simulink model "DBX_model_all"  (R2015a)
settings: Solver=ode2  SolverMode=SingleTasking  StartTime=0.0  StopTime=10.0  FixedStep=T_sim  RelTol=1e-3
values from neighbouring files (symbols this model uses):
  A_M = 2/sqrt(3)*L_M    [SetupComplete.m]    (also in simple_all.m = single(A_M))
  Alpha_unique_rad = deg2rad(Alpha_unique)    [DBX_aero_V1.m]    (also in simple_all.m = single(Alpha_unique_rad))
  as = aerosonde_data_mod    [SetupComplete.m]
  B_span = 3    [SetupComplete.m]    (also in simple_all.m = single(B_span))
  Beta_unique_rad = deg2rad(Beta_unique)    [DBX_aero_V1.m]    (also in simple_all.m = single(Beta_unique_rad))
  C_D_q = 0.0336    [DBX_aero_V1.m]    (also in simple_all.m = single(C_D_q))
  C_l = NaN*ones(size(Alpha_unique,1),size(Beta_unique,1) )    [DBX_aero_V1.m]    (also in simple_all.m = single(C_l))
  C_l_delta_a_Asim = C_l_raw(idx)/deg2rad(delta_ale(idx))    [DBX_aero_V1.m]    (also in simple_all.m = single(C_l_delta_a_Asim))
  C_l_delta_rv_Asim = C_l_raw(idx)/deg2rad(delta_rud(idx))    [DBX_aero_V1.m]    (also in simple_all.m = single(C_l_delta_rv_Asim))
  C_l_p = -0.8333    [DBX_aero_V1.m]    (also in simple_all.m = single(C_l_p))
  C_l_r = 0.0347    [DBX_aero_V1.m]    (also in simple_all.m = single(C_l_r))
  C_Lift_q = 10.9    [DBX_aero_V1.m]    (also in simple_all.m = single(C_Lift_q))
  C_m = NaN*ones(size(Alpha_unique,1),size(Beta_unique,1),size(delta_elev_unique,1) )    [DBX_aero_V1.m]    (also in simple_all.m = single(C_m))
  C_m_q = -45.7828    [DBX_aero_V1.m]    (also in simple_all.m = single(C_m_q))
  C_n = NaN*ones(size(Alpha_unique,1),size(Beta_unique,1) )    [DBX_aero_V1.m]    (also in simple_all.m = single(C_n))
  C_n_delta_a_Asim = C_n_raw(idx)/deg2rad(delta_ale(idx))    [DBX_aero_V1.m]    (also in simple_all.m = single(C_n_delta_a_Asim))
  C_n_delta_rv_Asim = C_n_raw(idx)/deg2rad(delta_rud(idx))    [DBX_aero_V1.m]    (also in simple_all.m = single(C_n_delta_rv_Asim))
  C_n_p = -0.0066    [DBX_aero_V1.m]    (also in simple_all.m = single(C_n_p))
  C_n_r = -0.1827    [DBX_aero_V1.m]    (also in simple_all.m = single(C_n_r))
  C_X = NaN*ones(size(Alpha_unique,1),size(Beta_unique,1),size(delta_elev_unique,1) )    [DBX_aero_V1.m]    (also in simple_all.m = single(C_X))
  C_Y = NaN*ones(size(Alpha_unique,1),size(Beta_unique,1) )    [DBX_aero_V1.m]    (also in simple_all.m = single(C_Y))
  C_Y_delta_rv_Asim = C_y(idx)/deg2rad(delta_rud(idx))    [DBX_aero_V1.m]    (also in simple_all.m = single(C_Y_delta_rv_Asim))
  C_Y_p = -0.0991    [DBX_aero_V1.m]    (also in simple_all.m = single(C_Y_p))
  C_Y_r = 0.5219    [DBX_aero_V1.m]    (also in simple_all.m = single(C_Y_r))
  C_Z = NaN*ones(size(Alpha_unique,1),size(Beta_unique,1),size(delta_elev_unique,1) )    [DBX_aero_V1.m]    (also in simple_all.m = single(C_Z))
  CG = (m_OE*CG_OE + m_PL*CG_PL)/m    [SetupComplete.m]    (also in simple_all.m = single(CG))
  CMA = 0.25    [SetupComplete.m]    (also in simple_all.m = single(CMA))
  delta_elev_unique_rad = deg2rad(delta_elev_unique)    [DBX_aero_V1.m]    (also in simple_all.m = single(delta_elev_unique_rad))
  g = 9.81    [SetupComplete.m]    (also in simple_all.m = single(g))
  h_1 = -0.0666    [SetupComplete.m]    (also in simple_all.m = single(h_1))
  h_2 = -0.0666    [SetupComplete.m]    (also in simple_all.m = single(h_2))
  h_3 = -0.04824    [SetupComplete.m]    (also in simple_all.m = single(h_3))
  I_BAC = I_CG + m*[CG(3)^2,0,CG(1)*CG(3);0,CG(1)^2+CG(3)^2,0;CG(1)*CG(3),0,CG(1)^2]    [SetupComplete.m]    (also in simple_all.m = single(I_BAC))
  Initial_Omegas = max(0,Omega_0)    [Run_DBX.m]    (also in simple_all.m = single(Initial_Omegas))
  Initial_Torques = Torque_0    [Run_DBX.m]    (also in simple_all.m = single(Initial_Torques))
  L_M = 1.20    (= 1.2)    [SetupComplete.m]    (also in simple_all.m = single(L_M))
  m = m_OE + m_PL    (= 14.5)    [SetupComplete.m]    (also in simple_all.m = single(m))
  Rotation_sign = [-1,-1,-1]    [SetupComplete.m]    (also in simple_all.m = single(Rotation_sign))
undefined symbols (not defined in the file or in its folder): DOWN_0, EAST_0, F, MIL, NORTH_0, P_0, Q_0, R_0, Servo_calib, U_0, V_0, W_0
libraries: DBX_model x14, aerolibwind2 x6, aerolibasang x5, aerolibadyn x2, aerolibtransform2 x1
(part 1 of 2)
settings Model: ExtModeTrigDuration=5000  Creator=DavidTorres  LastModifiedBy=David
settings DataIOCC: LimitDataPoints=off  SaveOutput=off  SignalLogging=off  DSMLogging=off  VisualizeSimOutput=off  SaveTime=off
settings OptimizationCC: InlineParams=on  UseDivisionForNetSlopeComputation=on  UseFloatMulNetSlope=on  InlineInvariantSignals=on  EfficientFloat2IntCast=on
settings DebuggingCC: AlgebraicLoopMsg=error  SaveWithParameterizedLinksMsg=none  UniqueDataStoreMsg=error  StrictBusMsg=ErrorOnBusTreatedAsVector
settings HardwareCC: ProdLargestAtomicInteger=Long  ProdLargestAtomicFloat=Double  ProdIntDivRoundTo=Zero  ProdEndianess=LittleEndian  ProdHWDeviceType=Generic->32-bit x86 compatible  TargetUnknown=on
settings ModelReferenceCC: ModelReferenceNumInstancesAllowed=Single  ModelReferencePassRootInputsByReference=off

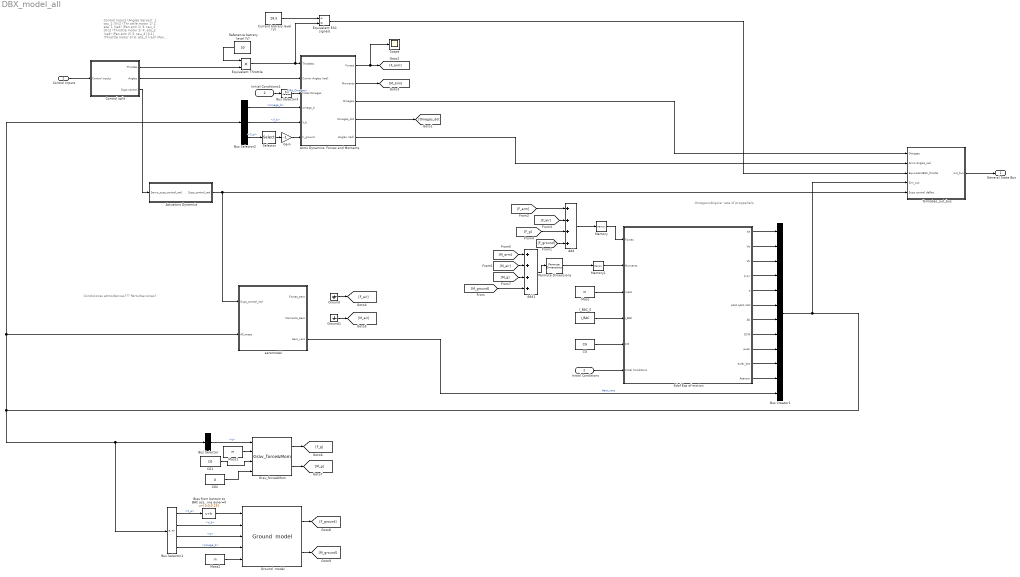
== system DBX_model_all ==
  note: Condiciones atmosfericas???
      | Perturbaciones?
  note: Omegas=Angular rate of proppellers
  note: Control inputs (Angles Servos):
      |
      | 1. tau_1 [0-1] (Thr ottle motor 1)
      | 2. eta_1 (rad)  (Pan arm 1)
      |
      | 3. tau_2 [0-1] (Throttle motor 2)
      | 4. eta_2 (rad)  (Pan arm 2)
      |
      | 5. tau_3 [0-1] (Throttle motor 3)
      | 6. eta_3 (rad)  (Pan arm  3)
      |
      | 7. Rudervator Left (rad)
      | 8. Rudervator Right (rad)
      | 9. Aileron Left (rad)
      | 10. Aielron Right (rad)
  Control Inputs : Inport
  Initial Conditions : Inport  Port=2  OutDataTypeStr=Bus: slBus1
  6dof Eqs of motion : Subsystem  TreatAsAtomicUnit=on
  Actuators Dynamcis : Subsystem  TreatAsAtomicUnit=on
  Add : Sum  Inputs=++++
  Add1 : Sum  Inputs=++++
  Arms Dynamics: Forces and Moments : Subsystem
  Bias from bottom to BAC assuming euler=0 : Bias  Bias=[0;0;0.25]
  Bus Creator1 : BusCreator  Inputs=12
  Bus Selector : BusSelector  OutputSignals=q
  Bus Selector1 : BusSelector  OutputSignals=X_e,V_b,q,omega_b
  Bus Selector2 : BusSelector  OutputSignals=omega_b,V_b,X_e
  Bus Selector3 : BusSelector  OutputSignals=Init_Omegas
  CG : Constant  Value=CG
  CG1 : Constant  Value=CG
  CG2 : Constant  Value=g
  Control split : Subsystem  TreatAsAtomicUnit=on
  Current batrery level (V) : Constant  Value=28.5
  Equivalent ESC signals : Product  Inputs=/*
  Equivalent Throttle : Product  Inputs=**
  Gain : Gain  Gain=-1
  Grav_force&Mom : DBX_model/Grav_force&Mom
  Ground : Ground
  Ground  model : DBX_model/Ground  model
  Ground1 : Ground
  I_BAC_0 : Constant  Value=I_BAC
  Initial Conditions1 : InportShadow  Port=2  OutDataTypeStr=Bus: slBus1
  Mass : Constant  Value=m
  Mass1 : Constant  Value=m
  Mass2 : Constant  Value=m
  Memory : Memory  X0=[0,0,0]'
  Memory1 : Memory  X0=[0,0,0]'
  Permute Dimensions : PermuteDimensions
  Reference batrery level (V) : Constant  Value=30
  Scope : Scope
      settings: TimeRange=100  YMin=-175  YMax=150
  Selector : Selector  InputPortWidth=3  Indices=3
  aeromodel : Subsystem  Variant=on  OverrideUsingVariant=AeroAerosonde
  formateo_out_bus : Subsystem
  General State Bus : Outport  OutDataTypeStr=Bus: slBus3
  wires:
  Initial Conditions/1 -> 6dof Eqs of motion/6(Initial Conditions)
  6dof Eqs of motion/3(Vb) -> Bus Creator1/3
  6dof Eqs of motion/5(q) -> Bus Creator1/5
  6dof Eqs of motion/2(Ve) -> Bus Creator1/2
  6dof Eqs of motion/6(pdot,qdot,rdot) -> Bus Creator1/6
  6dof Eqs of motion/1(Xe) -> Bus Creator1/1
  6dof Eqs of motion/7(Ab) -> Bus Creator1/7
  6dof Eqs of motion/8(DCM) -> Bus Creator1/8
  6dof Eqs of motion/9(euler) -> Bus Creator1/9
  6dof Eqs of motion/10(euler_dot) -> Bus Creator1/10
  Bus Selector/1 -> Grav_force&Mom/1  "<q>"
  Mass/1 -> 6dof Eqs of motion/3(mass)
  Bus Selector2/1 -> Arms Dynamics: Forces and Moments/4(omega_b)  "<omega_b>"
  Bus Selector2/2 -> Arms Dynamics: Forces and Moments/5(V_b)  "<V_b>"
  Mass1/1 -> Grav_force&Mom/2
  Arms Dynamics: Forces and Moments/4(Omegas_dot) -> [Omegas_dot]
  Initial Conditions1/1 -> Bus Selector3/1
  Bus Selector2/3 -> Selector/1  "<X_e>"
  Selector/1 -> Gain/1
  Gain/1 -> Arms Dynamics: Forces and Moments/6(h_ground)
  Arms Dynamics: Forces and Moments/1(Forces) -> Scope/1, [F_arm]
  Arms Dynamics: Forces and Moments/2(Moments) -> [M_arm]
  Grav_force&Mom/1 -> [F_g]
  Grav_force&Mom/2 -> [M_g]
  [F_arm] -> Add/1
  [F_air] -> Add/2
  [F_g] -> Add/3
  [M_arm] -> Add1/1
  [M_g] -> Add1/3
  [M_air] -> Add1/2
  6dof Eqs of motion/11(Asensor) -> Bus Creator1/11
  Control split/1("Throtles ") -> Equivalent Throttle/2
  Control split/2(Angles) -> Arms Dynamics: Forces and Moments/2(Comm Angles (rad))
  Arms Dynamics: Forces and Moments/3(Omegas) -> formateo_out_bus/1(Omegas)
  Memory/1 -> 6dof Eqs of motion/1(Forces)
  Memory1/1 -> 6dof Eqs of motion/2(Moments)
  CG/1 -> 6dof Eqs of motion/5(CG)
  I_BAC_0/1 -> 6dof Eqs of motion/4(I_BAC)
  Equivalent Throttle/1 -> Arms Dynamics: Forces and Moments/1(Throttles), Equivalent ESC signals/2
  Reference batrery level (V)/1 -> Equivalent Throttle/1
  Current batrery level (V)/1 -> Equivalent ESC signals/1
  Equivalent ESC signals/1 -> formateo_out_bus/3(EquivalentESC_throtle)
  6dof Eqs of motion/4(p,q,r) -> Bus Creator1/4
  Arms Dynamics: Forces and Moments/5(Angles (rad)) -> formateo_out_bus/2(Arms Angles_rad)
  Control Inputs/1 -> Control split/1(Control inputs)
  CG1/1 -> Grav_force&Mom/3
  Control split/3(Sups control) -> Actuators Dynamcis/1(Servo_sups_control_rad)
  formateo_out_bus/1(out_bus) -> General State Bus/1
  Bus Selector3/1 -> Arms Dynamics: Forces and Moments/3(Initial Omegas)  "<Init_Omegas>"
  Actuators Dynamcis/1(Sups_control_rad) -> aeromodel/1(Sups_control_rad), formateo_out_bus/5(Sups control deflec)
  Add/1 -> Memory/1
  Add1/1 -> Permute Dimensions/1
  aeromodel/3(Aero_vars) -> Bus Creator1/12  "Aero_vars"
  Permute Dimensions/1 -> Memory1/1
  Ground/1 -> [F_air]
  Ground1/1 -> [M_air]
  Bus Creator1/1 -> formateo_out_bus/4(Sim_out), Bus Selector1/1, Bus Selector/1, Bus Selector2/1, aeromodel/2(All_meas)
  Ground  model/1 -> [F_ground]
  Ground  model/2 -> [M_ground]
  Bus Selector1/1 -> Bias from bottom to BAC assuming euler=0/1  "<X_e>"
  Bus Selector1/3 -> Ground  model/3  "<q>"
  Mass2/1 -> Ground  model/5
  Bus Selector1/2 -> Ground  model/2  "<V_b>"
  Bus Selector1/4 -> Ground  model/4  "<omega_b>"
  Bias from bottom to BAC assuming euler=0/1 -> Ground  model/1
  CG2/1 -> Grav_force&Mom/4
  [M_ground] -> Add1/4
  [F_ground] -> Add/4

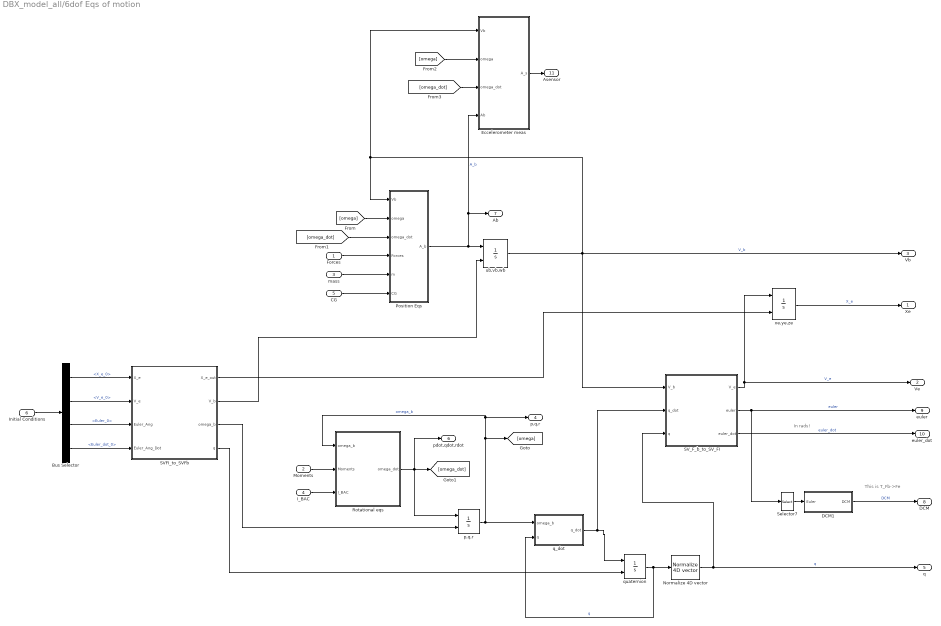
== system DBX_model_all/6dof Eqs of motion ==
  note: In rads!
  note: This is T_Fb->Fe
  Forces : Inport
  Moments : Inport  Port=2
  mass : Inport  Port=3
  I_BAC : Inport  Port=4
  CG : Inport  Port=5
  Initial Conditions : Inport  Port=6
  Bus Selector : BusSelector  OutputSignals=X_e_0,V_e_0,Euler_0,Euler_dot_0
  DCM1 : Subsystem  TreatAsAtomicUnit=on
  Eccelerometer meas : MATLAB Function  TreatAsAtomicUnit=on
  Normalize 4D vector : DBX_model/Normalize 4D vector
  Position Eqs : MATLAB Function  TreatAsAtomicUnit=on
  Rotational eqs : MATLAB Function  TreatAsAtomicUnit=on
  SVFI_to_SVFb : MATLAB Function  TreatAsAtomicUnit=on
  SV_F_b_to_SV_FI : MATLAB Function  TreatAsAtomicUnit=on
  Selector7 : Selector  InputPortWidth=3  Indices=[3 2 1]
  "p,q,r " : Integrator  InitialConditionSource=external  InitialCondition=[P_0,Q_0,R_0]
  q_dot : Subsystem  TreatAsAtomicUnit=on
  quaternion : Integrator  InitialConditionSource=external  InitialCondition=[P_0,Q_0,R_0]
  ub,vb,wb : Integrator  InitialConditionSource=external  InitialCondition=[U_0,V_0,W_0]
  xe,ye,ze : Integrator  InitialConditionSource=external  InitialCondition=[NORTH_0,EAST_0,-DOWN_0]
  Xe : Outport
  Ve : Outport  Port=2
  Vb : Outport  Port=3
  p,q,r : Outport  Port=4
  q : Outport  Port=5
  pdot,qdot,rdot : Outport  Port=6
  Ab : Outport  Port=7
  DCM : Outport  Port=8
  euler : Outport  Port=9
  euler_dot : Outport  Port=10
  Asensor : Outport  Port=11
  wires:
  I_BAC/1 -> Rotational eqs/3(I_BAC)
  mass/1 -> Position Eqs/5(m)
  Forces/1 -> Position Eqs/4(Forces)
  xe,ye,ze/1 -> Xe/1  "X_e"
  ub,vb,wb/1 -> Eccelerometer meas/1(Vb), Position Eqs/1(Vb), Vb/1, SV_F_b_to_SV_FI/1(V_b)  "V_b"
  SV_F_b_to_SV_FI/1(V_e) -> Ve/1, xe,ye,ze/1  "V_e"
  [omega] -> Position Eqs/2(omega)
  [omega_dot] -> Position Eqs/3(omega_dot)
  Position Eqs/1(A_b) -> Eccelerometer meas/4(Ab), Ab/1, ub,vb,wb/1  "A_b"
  CG/1 -> Position Eqs/6(CG)
  Initial Conditions/1 -> Bus Selector/1
  Bus Selector/1 -> SVFI_to_SVFb/1(X_e)  "<X_e_0>"
  Bus Selector/2 -> SVFI_to_SVFb/2(V_e)  "<V_e_0>"
  Bus Selector/3 -> SVFI_to_SVFb/3(Euler_Ang)  "<Euler_0>"
  Bus Selector/4 -> SVFI_to_SVFb/4(Euler_Ang_Dot)  "<Euler_dot_0>"
  SVFI_to_SVFb/2(V_b) -> ub,vb,wb/2
  SVFI_to_SVFb/1(X_e_out) -> xe,ye,ze/2
  SVFI_to_SVFb/3(omega_b) -> "p,q,r "/2
  Rotational eqs/1(omega_dot) -> pdot,qdot,rdot/1, [omega_dot], "p,q,r "/1
  "p,q,r "/1 -> q_dot/1(omega_b), [omega], p,q,r/1, Rotational eqs/1(omega_b)  "omega_b"
  q_dot/1(q_dot) -> quaternion/1, SV_F_b_to_SV_FI/2(q_dot)
  SVFI_to_SVFb/4(q) -> quaternion/2
  quaternion/1 -> Normalize 4D vector/1, q_dot/2(q)  "q"
  DCM1/1(DCM) -> DCM/1  "DCM"
  SV_F_b_to_SV_FI/2(euler) -> Selector7/1, euler/1  "euler"
  SV_F_b_to_SV_FI/3(euler_dot) -> euler_dot/1  "euler_dot"
  Moments/1 -> Rotational eqs/2(Moments)
  Normalize 4D vector/1 -> q/1, SV_F_b_to_SV_FI/3(q)  "q"
  [omega] -> Eccelerometer meas/2(omega)
  [omega_dot] -> Eccelerometer meas/3(omega_dot)
  Eccelerometer meas/1(A_s) -> Asensor/1
  Selector7/1 -> DCM1/1(Euler)

== system DBX_model_all/Actuators Dynamcis ==
  note: Relaciones no lineales aqui
  note: Control inputs:
      |
      |
      | 7. Rudervator Left (rad)
      | 8. Rudervator Right (rad)
      | 9. Aileron Left (rad)
      | 10. Aielron Right (rad)
  Servo_sups_control_rad : Inport
  Demux : Demux
  Mux2 : Mux
  Servo 1st order : DBX_model/Servo 1st order  Init_def=delta_rv_L_0_servo  Max_rate=6.159  Min_rate=-6.159  Max_defle=deg2rad(25)  Min_def=-deg2rad(25)  RT=0.01
  Servo 1st order1 : DBX_model/Servo 1st order  Init_def=delta_rv_R_0_servo  Max_rate=6.159  Min_rate=-6.159  Max_defle=deg2rad(25)  Min_def=-deg2rad(25)  RT=0.01
  Servo 1st order2 : DBX_model/Servo 1st order  Init_def=delta_a_L_0_servo  Max_rate=6.159  Min_rate=-6.159  Max_defle=deg2rad(25)  Min_def=-deg2rad(25)  RT=0.01
  Servo 1st order3 : DBX_model/Servo 1st order  Init_def=delta_a_R_0_servo  Max_rate=6.159  Min_rate=-6.159  Max_defle=deg2rad(25)  Min_def=-deg2rad(25)  RT=0.01
  Servo2Sup Lin conversion : DBX_model/Servo2Sup Lin conversion  Gain=Servo_calib.Servo4.Pendiente_Sup_Servo  Bias=Servo_calib.Servo4.Sup_rad_0
  Servo2Sup Lin conversion1 : DBX_model/Servo2Sup Lin conversion  Gain=Servo_calib.Servo5.Pendiente_Sup_Servo  Bias=Servo_calib.Servo5.Sup_rad_0
  Servo2Sup Lin conversion2 : DBX_model/Servo2Sup Lin conversion  Gain=Servo_calib.Servo6.Pendiente_Sup_Servo  Bias=Servo_calib.Servo6.Sup_rad_0
  Servo2Sup Lin conversion3 : DBX_model/Servo2Sup Lin conversion  Gain=Servo_calib.Servo7.Pendiente_Sup_Servo  Bias=Servo_calib.Servo7.Sup_rad_0
  Sups_control_rad : Outport
  wires:
  Servo_sups_control_rad/1 -> Demux/1
  Mux2/1 -> Sups_control_rad/1
  Demux/1 -> Servo 1st order/1
  Demux/2 -> Servo 1st order1/1
  Demux/3 -> Servo 1st order2/1
  Demux/4 -> Servo 1st order3/1
  Servo2Sup Lin conversion/1 -> Mux2/1
  Servo2Sup Lin conversion1/1 -> Mux2/2
  Servo2Sup Lin conversion2/1 -> Mux2/3
  Servo2Sup Lin conversion3/1 -> Mux2/4
  Servo 1st order/1 -> Servo2Sup Lin conversion/1
  Servo 1st order1/1 -> Servo2Sup Lin conversion1/1
  Servo 1st order2/1 -> Servo2Sup Lin conversion2/1
  Servo 1st order3/1 -> Servo2Sup Lin conversion3/1

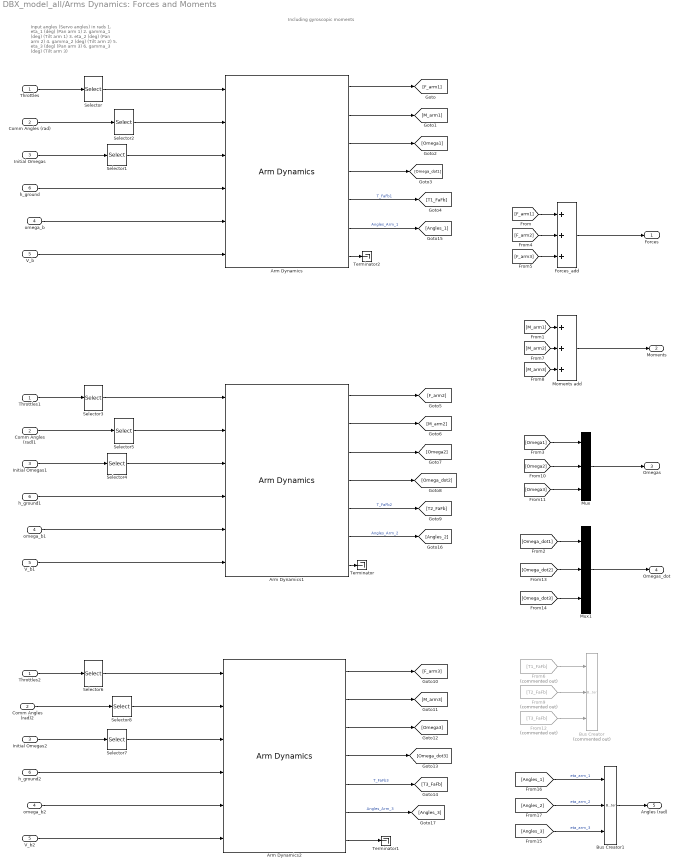
== system DBX_model_all/Arms Dynamics: Forces and Moments ==
  note: Including gyroscopic moments
  note: Input angles (Servo angles)  in rads
      |
      | 1. eta_1 (deg)  (Pan arm 1)
      | 2. gamma_1 (deg)  (Tilt arm 1)
      |
      | 3. eta_2 (deg)  (Pan arm 2)
      | 4. gamma_2 (deg)  (Tilt arm 2)
      |
      | 5. eta_3 (deg)  (Pan arm  3)
      | 6. gamma_3 (deg)  (Tilt arm 3)
  Throttles : Inport
  Comm Angles (rad) : Inport  Port=2
  Initial Omegas : Inport  Port=3
  omega_b : Inport  Port=4
  V_b : Inport  Port=5
  h_ground : Inport  Port=6
  Arm Dynamics : DBX_model/Arm Dynamics  arm_num=1  Rot_sign=Rotation_sign(1)  Hub_pos=[1/3*L_M;-A_M/2;h_1]  h_p=hp_1  Gain=[0;1;0]  UpperLimit=deg2rad(10)  LowerLimit=-deg2rad(90)  J_FA=J_FA_1  Inertia_swithc_var=None  Freno_param=Activo  J_T=J_T  tau=Tau_motors  Initi_omega=Initial_Omegas(1)  Init_torque=Initial_Torques(1)  omega_n=40  xi=1.45  init_eta=eta_1_0_servo  Gain_servos=Servo_calib.Servo1.Pendiente_Sup_Servo  Bias=Servo_calib.Servo1.Sup_rad_0
  Arm Dynamics1 : DBX_model/Arm Dynamics  arm_num=2  Rot_sign=Rotation_sign(2)  Hub_pos=[1/3*L_M;A_M/2;h_2]  h_p=hp_2  Gain=[0;1;0]  UpperLimit=deg2rad(10)  LowerLimit=-deg2rad(90)  J_FA=J_FA_2  Inertia_swithc_var=None  Freno_param=Activo  J_T=J_T  tau=Tau_motors  Initi_omega=Initial_Omegas(2)  Init_torque=Initial_Torques(2)  omega_n=40  xi=1.45  init_eta=eta_2_0_servo  Gain_servos=Servo_calib.Servo2.Pendiente_Sup_Servo  Bias=Servo_calib.Servo2.Sup_rad_0
  Arm Dynamics2 : DBX_model/Arm Dynamics  arm_num=3  Rot_sign=Rotation_sign(3)  Hub_pos=[-2/3*L_M;0;h_3]  h_p=hp_3  Gain=[1;0;0]  UpperLimit=deg2rad(60)  LowerLimit=-deg2rad(60)  J_FA=J_FA_3  Inertia_swithc_var=None  Freno_param=Activo  J_T=J_T  tau=Tau_motors  Initi_omega=Initial_Omegas(3)  Init_torque=Initial_Torques(3)  omega_n=40  xi=1.45  init_eta=eta_3_0  Gain_servos=Servo_calib.Servo3.Pendiente_Sup_Servo  Bias=Servo_calib.Servo3.Sup_rad_0
  Bus Creator : BusCreator  Commented=on  Inputs=3
  Bus Creator1 : BusCreator  Inputs=3
  Comm Angles (rad)1 : InportShadow  Port=2
  Comm Angles (rad)2 : InportShadow  Port=2
  Forces_add : Sum  Inputs=+++
  From12 : From  Commented=on  GotoTag=T3_FaFb
  From6 : From  Commented=on  GotoTag=T1_FaFb
  From9 : From  Commented=on  GotoTag=T2_FaFb
  Initial Omegas1 : InportShadow  Port=3
  Initial Omegas2 : InportShadow  Port=3
  Moments add : Sum  Inputs=+++
  Mux : Mux  Inputs=3
  Mux1 : Mux  Inputs=3
  Selector : Selector  InputPortWidth=3  Indices=[1]
  Selector1 : Selector  InputPortWidth=3  Indices=[1]
  Selector2 : Selector  InputPortWidth=3
  Selector3 : Selector  InputPortWidth=3  Indices=2
  Selector4 : Selector  InputPortWidth=3  Indices=2
  Selector5 : Selector  InputPortWidth=3  Indices=2
  Selector6 : Selector  InputPortWidth=3  Indices=3
  Selector7 : Selector  InputPortWidth=3  Indices=3
  Selector8 : Selector  InputPortWidth=3  Indices=3
  Terminator : Terminator
  Terminator1 : Terminator
  Terminator2 : Terminator
  Throttles1 : InportShadow
  Throttles2 : InportShadow
  V_b1 : InportShadow  Port=5
  V_b2 : InportShadow  Port=5
  h_ground1 : InportShadow  Port=6
  h_ground2 : InportShadow  Port=6
  omega_b1 : InportShadow  Port=4
  omega_b2 : InportShadow  Port=4
  Forces : Outport
  Moments : Outport  Port=2
  Omegas : Outport  Port=3
  Omegas_dot : Outport  Port=4
  Angles (rad) : Outport  Port=5
  wires:
  Selector1/1 -> Arm Dynamics/3
  Throttles/1 -> Selector/1
  Initial Omegas/1 -> Selector1/1
  Selector/1 -> Arm Dynamics/1
  V_b/1 -> Arm Dynamics/6
  Forces_add/1 -> Forces/1
  Moments add/1 -> Moments/1
  Mux/1 -> Omegas/1
  Mux1/1 -> Omegas_dot/1
  h_ground/1 -> Arm Dynamics/4
  Arm Dynamics/1 -> [F_arm1]
  Arm Dynamics/2 -> [M_arm1]
  Arm Dynamics/3 -> [Omega1]
  Arm Dynamics/4 -> [Omega_dot1]
  [F_arm1] -> Forces_add/1
  [M_arm1] -> Moments add/1
  [Omega_dot1] -> Mux1/1
  [Omega1] -> Mux/1
  omega_b/1 -> Arm Dynamics/5
  [F_arm2] -> Forces_add/2
  [F_arm3] -> Forces_add/3
  [Omega2] -> Mux/2
  [Omega3] -> Mux/3
  [Omega_dot2] -> Mux1/2
  [Omega_dot3] -> Mux1/3
  [M_arm3] -> Moments add/3
  [M_arm2] -> Moments add/2
  Selector2/1 -> Arm Dynamics/2
  Comm Angles (rad)/1 -> Selector2/1
  Arm Dynamics/5 -> [T1_FaFb]  "T_FaFb1"
  From6/1 -> Bus Creator/1
  Selector4/1 -> Arm Dynamics1/3
  Throttles1/1 -> Selector3/1
  Initial Omegas1/1 -> Selector4/1
  Selector3/1 -> Arm Dynamics1/1
  V_b1/1 -> Arm Dynamics1/6
  h_ground1/1 -> Arm Dynamics1/4
  Arm Dynamics1/1 -> [F_arm2]
  Arm Dynamics1/2 -> [M_arm2]
  Arm Dynamics1/3 -> [Omega2]
  Arm Dynamics1/4 -> [Omega_dot2]
  omega_b1/1 -> Arm Dynamics1/5
  Selector5/1 -> Arm Dynamics1/2
  Comm Angles (rad)1/1 -> Selector5/1
  Arm Dynamics1/5 -> [T2_FaFb]  "T_FaFb2"
  From9/1 -> Bus Creator/2
  Selector7/1 -> Arm Dynamics2/3
  Throttles2/1 -> Selector6/1
  Initial Omegas2/1 -> Selector7/1
  Selector6/1 -> Arm Dynamics2/1
  V_b2/1 -> Arm Dynamics2/6
  h_ground2/1 -> Arm Dynamics2/4
  Arm Dynamics2/1 -> [F_arm3]
  Arm Dynamics2/2 -> [M_arm3]
  Arm Dynamics2/3 -> [Omega3]
  Arm Dynamics2/4 -> [Omega_dot3]
  omega_b2/1 -> Arm Dynamics2/5
  Selector8/1 -> Arm Dynamics2/2
  Comm Angles (rad)2/1 -> Selector8/1
  Arm Dynamics2/5 -> [T3_FaFb]  "T_FaFb3"
  From12/1 -> Bus Creator/3
  Bus Creator1/1 -> Angles (rad)/1
  [Angles_1] -> Bus Creator1/1  "eta_arm_1"
  [Angles_2] -> Bus Creator1/2  "eta_arm_2"
  [Angles_3] -> Bus Creator1/3  "eta_arm_3"
  Arm Dynamics/6 -> [Angles_1]  "Angles_Arm_1"
  Arm Dynamics1/6 -> [Angles_2]  "Angles_Arm_2"
  Arm Dynamics2/6 -> [Angles_3]  "Angles_Arm_3"
  Arm Dynamics1/7 -> Terminator/1
  Arm Dynamics2/7 -> Terminator1/1
  Arm Dynamics/7 -> Terminator2/1

== system DBX_model_all/Control split ==
  Control inputs : Inport
  Saturation : Saturate  UpperLimit=1  LowerLimit=0
  Throttles : Selector  InputPortWidth=10  Indices=[1,3,5]
  Throttles1 : Selector  InputPortWidth=10  Indices=[2,4,6]
  Throttles2 : Selector  InputPortWidth=10  Indices=[7:10]
  "Throtles " : Outport
  Angles : Outport  Port=2
  Sups control : Outport  Port=3
  wires:
  Control inputs/1 -> Throttles2/1, Throttles1/1, Throttles/1
  Throttles/1 -> Saturation/1
  Throttles1/1 -> Angles/1
  Saturation/1 -> "Throtles "/1
  Throttles2/1 -> Sups control/1

== system DBX_model_all/aeromodel ==
  note: 1) Add Subsystem or Model blocks as valid variant choices.
      | 2) You cannot connect blocks at this level. At simulation, connectivity is automatically
      | determined, based on the active variant and port name matching.
  Sups_control_rad : Inport
  All_meas : Inport  Port=2
  Aero model : Subsystem  VariantControl=AeroDavid
  Aero model aerosonde : Subsystem  VariantControl=AeroAerosonde
  Forces_aero : Outport
  Moments_Aero : Outport  Port=2
  Aero_vars : Outport  Port=3

== system DBX_model_all/formateo_out_bus ==
  Omegas : Inport
  Arms Angles_rad : Inport  Port=2
  EquivalentESC_throtle : Inport  Port=3
  Sim_out : Inport  Port=4
  Sups control deflec : Inport  Port=5
  Bus Selector3 : BusSelector  OutputSignals=X_e,V_e,V_b,omega_b,q,omega_dot,A_b,DCM,euler,euler_dot,A_s,Aero_vars
  Bus Creator2 : BusCreator  Inputs=16  OutDataTypeStr=Bus: slBus3  NonVirtualBus=on
  Reshape : Reshape
  out_bus : Outport
  wires:
  Bus Selector3/6 -> Bus Creator2/6  "<omega_dot>"
  Bus Creator2/1 -> out_bus/1
  Bus Selector3/9 -> Bus Creator2/9  "<euler>"
  Bus Selector3/4 -> Bus Creator2/4  "<omega_b>"
  Bus Selector3/3 -> Bus Creator2/3  "<V_b>"
  Bus Selector3/7 -> Bus Creator2/7  "<A_b>"
  Bus Selector3/10 -> Bus Creator2/10  "<euler_dot>"
  Bus Selector3/5 -> Bus Creator2/5  "<q>"
  Bus Selector3/8 -> Reshape/1  "<DCM>"
  Bus Selector3/1 -> Bus Creator2/1  "<X_e>"
  Bus Selector3/11 -> Bus Creator2/11  "<A_s>"
  Bus Selector3/2 -> Bus Creator2/2  "<V_e>"
  Sim_out/1 -> Bus Selector3/1
  Reshape/1 -> Bus Creator2/8  "DCM_Vect"
  Omegas/1 -> Bus Creator2/13  "Omegas"
  Arms Angles_rad/1 -> Bus Creator2/14  "Ang_arms_rad"
  EquivalentESC_throtle/1 -> Bus Creator2/15  "EquivalentESC_throtle"
  Sups control deflec/1 -> Bus Creator2/16  "Sups_control_defl"
  Bus Selector3/12 -> Bus Creator2/12  "<Aero_vars>"

== system DBX_model_all/6dof Eqs of motion/DCM1 ==
  Euler : Inport  PortDimensions=3
  Fcn11 : Fcn  Expr=u(5)*u(4)
  Fcn12 : Fcn  Expr=u(5)*u(1)
  Fcn13 : Fcn  Expr=-u(2)
  Fcn21 : Fcn  Expr=u(3)*u(2)*u(4) - u(6)*u(1)
  Fcn22 : Fcn  Expr=u(3)*u(2)*u(1) + u(6)*u(4)
  Fcn23 : Fcn  Expr=u(3)*u(5)
  Fcn31 : Fcn  Expr=u(6)*u(2)*u(4) + u(3)*u(1)
  Fcn32 : Fcn  Expr=u(6)*u(2)*u(1) - u(3)*u(4)
  Fcn33 : Fcn  Expr=u(6)*u(5)
  Mux : Mux  Inputs=2
  Mux1 : Mux  Inputs=9
  Reshape : Reshape  OutputDimensionality=Customize  OutputDimensions=[3,3]
  sincos : Trigonometry  Operator=sincos
  DCM : Outport  PortDimensions=[3,3]
  wires:
  Fcn33/1 -> Mux1/9
  Fcn32/1 -> Mux1/8
  Fcn23/1 -> Mux1/6
  Fcn22/1 -> Mux1/5
  Fcn31/1 -> Mux1/7
  Fcn21/1 -> Mux1/4
  Fcn13/1 -> Mux1/3
  Fcn12/1 -> Mux1/2
  Fcn11/1 -> Mux1/1
  Mux/1 -> Fcn22/1, Fcn23/1, Fcn31/1, Fcn33/1, Fcn32/1, Fcn21/1, Fcn13/1, Fcn12/1, Fcn11/1
  sincos/2 -> Mux/2
  sincos/1 -> Mux/1
  Reshape/1 -> DCM/1
  Euler/1 -> sincos/1
  Mux1/1 -> Reshape/1

== system DBX_model_all/6dof Eqs of motion/q_dot ==
  note: Both of these methods to compute q_dot are very similar
  omega_b : Inport
  q : Inport  Port=2
  Quaternion_dot : MATLAB Function  TreatAsAtomicUnit=on  VariantControl=Variant
  q_dot : Outport
  wires:
  omega_b/1 -> Quaternion_dot/1(omega_b)  "omega_b"
  q/1 -> Quaternion_dot/2(q)  "q"
  Quaternion_dot/1(q_dot) -> q_dot/1

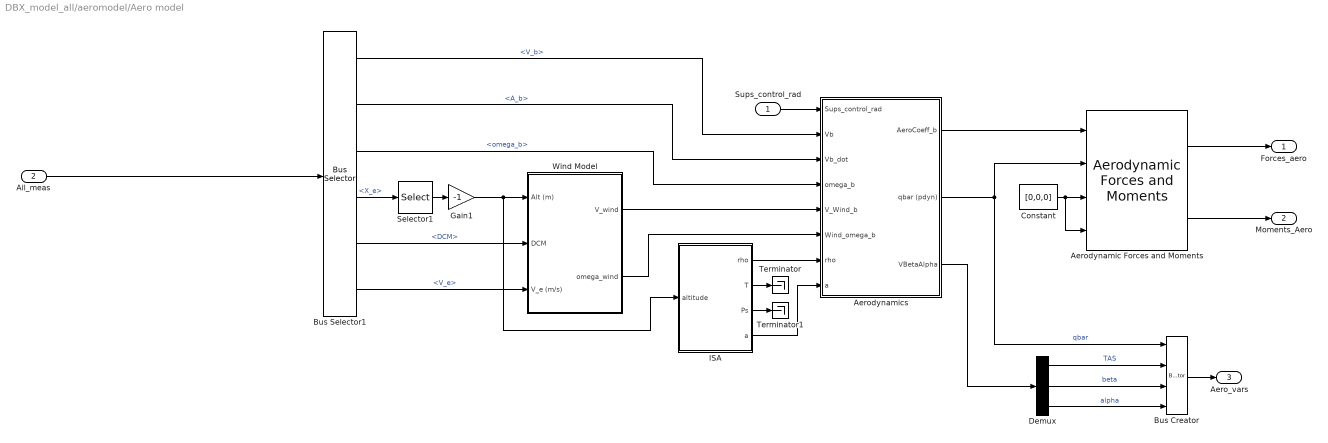
== system DBX_model_all/aeromodel/Aero model ==
  Sups_control_rad : Inport
  All_meas : Inport  Port=2
  Aerodynamic Forces and Moments : aerolibadyn/Aerodynamic Forces and Moments   inputAxes=Body  outputForceAxes=Body  outputMomentAxes=Body  S=S_w  b=B_span  cbar=CMA
  Aerodynamics : Subsystem
  Bus Creator : BusCreator
  Bus Selector1 : BusSelector  OutputSignals=V_b,A_b,omega_b,X_e,DCM,V_e
  Constant : Constant  Value=[0,0,0]
  Demux : Demux  Outputs=3
  Gain1 : Gain  Gain=-1
  ISA : MATLAB Function  TreatAsAtomicUnit=on
  Selector1 : Selector  InputPortWidth=3  Indices=3
  Terminator : Terminator
  Terminator1 : Terminator
  Wind Model : Subsystem
  Forces_aero : Outport
  Moments_Aero : Outport  Port=2
  Aero_vars : Outport  Port=3
  wires:
  All_meas/1 -> Bus Selector1/1
  Sups_control_rad/1 -> Aerodynamics/1(Sups_control_rad)
  Bus Selector1/1 -> Aerodynamics/2(Vb)  "<V_b>"
  Selector1/1 -> Gain1/1
  Bus Selector1/4 -> Selector1/1  "<X_e>"
  Gain1/1 -> ISA/1(altitude), Wind Model/1(Alt (m))
  Bus Selector1/5 -> Wind Model/2(DCM)  "<DCM>"
  Bus Selector1/6 -> Wind Model/3(V_e (m/s))  "<V_e>"
  Wind Model/1(V_wind) -> Aerodynamics/5(V_Wind_b)
  Bus Selector1/2 -> Aerodynamics/3(Vb_dot)  "<A_b>"
  Bus Selector1/3 -> Aerodynamics/4(omega_b)  "<omega_b>"
  Wind Model/2(omega_wind) -> Aerodynamics/6(Wind_omega_b)
  ISA/4(a) -> Aerodynamics/8("a ")
  ISA/1(rho) -> Aerodynamics/7(rho)
  Aerodynamics/2(qbar (pdyn)) -> Bus Creator/1, Aerodynamic Forces and Moments/2  "qbar"
  ISA/2(T) -> Terminator/1
  ISA/3(Ps) -> Terminator1/1
  Constant/1 -> Aerodynamic Forces and Moments/4, Aerodynamic Forces and Moments/3
  Aerodynamics/1(AeroCoeff_b) -> Aerodynamic Forces and Moments/1
  Aerodynamic Forces and Moments/1 -> Forces_aero/1
  Aerodynamic Forces and Moments/2 -> Moments_Aero/1
  Demux/2 -> Bus Creator/3  "beta"
  Demux/3 -> Bus Creator/4  "alpha"
  Bus Creator/1 -> Aero_vars/1
  Demux/1 -> Bus Creator/2  "TAS"
  Aerodynamics/3(VBetaAlpha) -> Demux/1

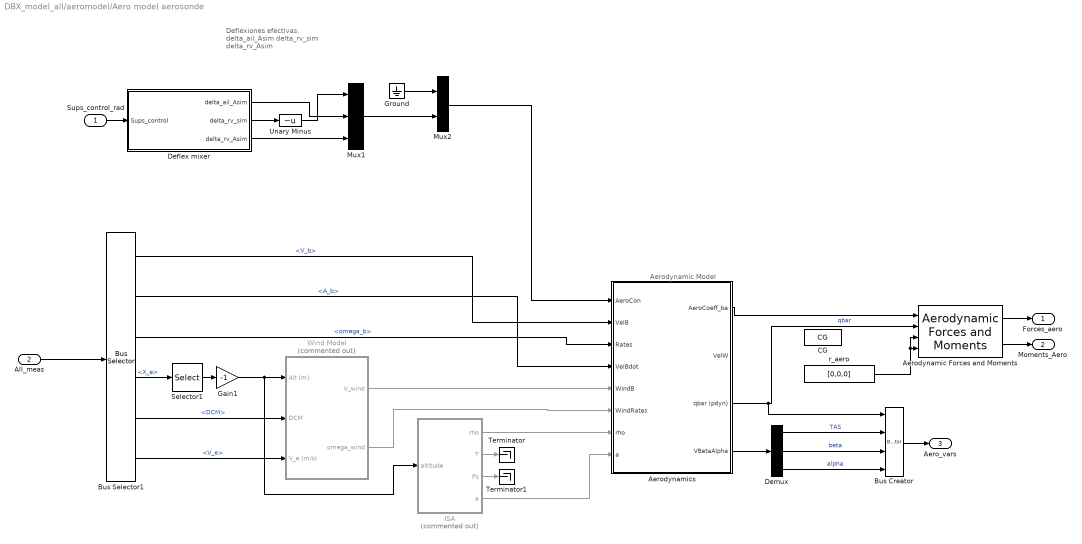
== system DBX_model_all/aeromodel/Aero model aerosonde ==
  note: Aerodynamic Model
  note: Deflexiones efectivas:
      |
      | delta_ail_Asim
      | delta_rv_sim
      | delta_rv_Asim
  Sups_control_rad : Inport
  All_meas : Inport  Port=2
  Aerodynamic Forces and Moments : aerolibadyn/Aerodynamic Forces and Moments   inputAxes=Body  outputForceAxes=Body  outputMomentAxes=Body  S=S_w  b=B_span  cbar=CMA
  Aerodynamics : Subsystem
  Bus Creator : BusCreator
  Bus Selector1 : BusSelector  OutputSignals=V_b,A_b,omega_b,X_e,DCM,V_e
  CG : Constant  Value=CG
  Deflex mixer : Subsystem  TreatAsAtomicUnit=on
  Demux : Demux  Outputs=3
  Gain1 : Gain  Gain=-1
  Ground : Ground
  ISA : MATLAB Function  Commented=on  TreatAsAtomicUnit=on
  Mux1 : Mux  Inputs=3
  Mux2 : Mux  Inputs=[1,3]
  Selector1 : Selector  InputPortWidth=3  Indices=3
  Terminator : Terminator
  Terminator1 : Terminator
  Unary Minus : UnaryMinus
  Wind Model : Subsystem  Commented=on
  r_aero : Constant  Value=[0,0,0]
  Forces_aero : Outport
  Moments_Aero : Outport  Port=2
  Aero_vars : Outport  Port=3
  wires:
  Aerodynamic Forces and Moments/2 -> Moments_Aero/1
  Aerodynamic Forces and Moments/1 -> Forces_aero/1
  r_aero/1 -> Aerodynamic Forces and Moments/3, Aerodynamic Forces and Moments/4
  Aerodynamics/1(AeroCoeff_ba) -> Aerodynamic Forces and Moments/1
  Aerodynamics/3(qbar (pdyn)) -> Bus Creator/1, Aerodynamic Forces and Moments/2  "qbar"
  All_meas/1 -> Bus Selector1/1
  Sups_control_rad/1 -> Deflex mixer/1(Sups_control)
  Bus Selector1/1 -> Aerodynamics/2(VelB)  "<V_b>"
  Selector1/1 -> Gain1/1
  Bus Selector1/4 -> Selector1/1  "<X_e>"
  Gain1/1 -> ISA/1(altitude), Wind Model/1(Alt (m))
  Bus Selector1/5 -> Wind Model/2(DCM)  "<DCM>"
  Bus Selector1/6 -> Wind Model/3(V_e (m/s))  "<V_e>"
  Wind Model/1(V_wind) -> Aerodynamics/5(WindB)
  Bus Selector1/2 -> Aerodynamics/4(VelBdot)  "<A_b>"
  Bus Selector1/3 -> Aerodynamics/3(Rates)  "<omega_b>"
  Wind Model/2(omega_wind) -> Aerodynamics/6(WindRates)
  ISA/4(a) -> Aerodynamics/8("a ")
  ISA/1(rho) -> Aerodynamics/7(rho)
  ISA/2(T) -> Terminator/1
  ISA/3(Ps) -> Terminator1/1
  Mux1/1 -> Mux2/2
  Ground/1 -> Mux2/1
  Deflex mixer/2(delta_rv_sim) -> Unary Minus/1
  Deflex mixer/3(delta_rv_Asim) -> Mux1/3
  Mux2/1 -> Aerodynamics/1(AeroCon)
  Unary Minus/1 -> Mux1/1
  Bus Creator/1 -> Aero_vars/1
  Aerodynamics/4(VBetaAlpha) -> Demux/1
  Demux/1 -> Bus Creator/2  "TAS"
  Demux/2 -> Bus Creator/3  "beta"
  Demux/3 -> Bus Creator/4  "alpha"
  Deflex mixer/1(delta_ail_Asim) -> Mux1/2

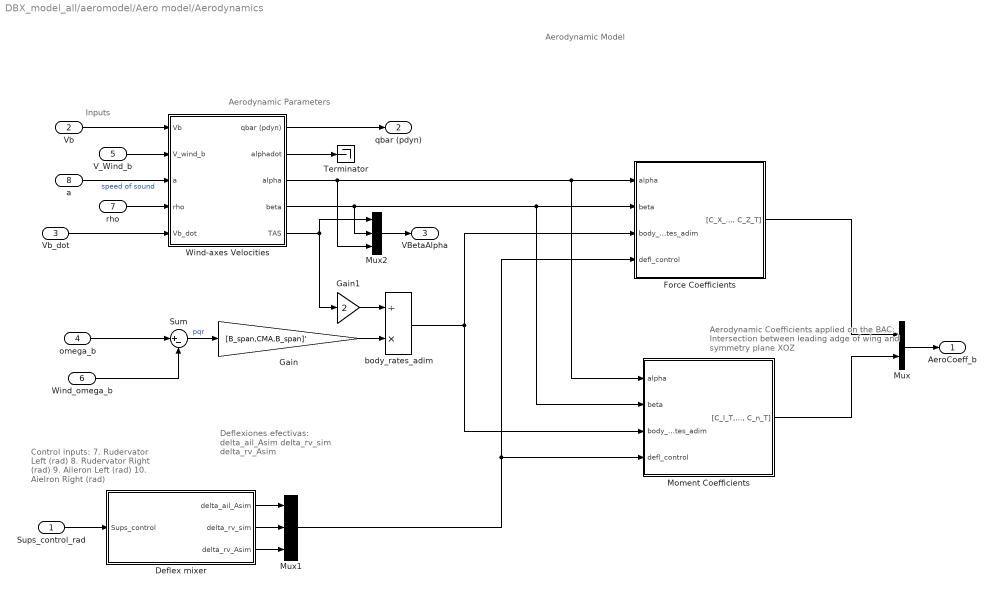
== system DBX_model_all/aeromodel/Aero model/Aerodynamics ==
  note: Deflexiones efectivas:
      |
      | delta_ail_Asim
      | delta_rv_sim
      | delta_rv_Asim
  note: Aerodynamic Model
  note: Aerodynamic Coefficients applied on the BAC:
      |
      | Intersection between leading adge of wing and
      | symmetry plane XOZ
  note: Aerodynamic Parameters
  note: Inputs
  note: Control inputs:
      |
      | 7. Rudervator Left (rad)
      | 8. Rudervator Right (rad)
      | 9. Aileron Left (rad)
      | 10. Aielron Right (rad)
  Sups_control_rad : Inport  PortDimensions=[4 1]
  Vb : Inport  Port=2  PortDimensions=[3 1]
  Vb_dot : Inport  Port=3
  omega_b : Inport  Port=4  PortDimensions=[3 1]
  V_Wind_b : Inport  Port=5  PortDimensions=[3 1]
  Wind_omega_b : Inport  Port=6  PortDimensions=[3 1]
  rho : Inport  Port=7  PortDimensions=1
  "a " : Inport  Port=8  PortDimensions=1
  Deflex mixer : Subsystem  TreatAsAtomicUnit=on
  Force Coefficients : Subsystem
  Gain : Gain  Gain=[B_span,CMA,B_span]'
  Gain1 : Gain  Gain=2
  Moment Coefficients : Subsystem
  Mux : Mux  Inputs=2
  Mux1 : Mux  Inputs=3
  Mux2 : Mux  Inputs=3
  Sum : Sum  Inputs=|+-  SaturateOnIntegerOverflow=on  InputSameDT=on  OutDataTypeStr=Inherit: Same as first input
  Terminator : Terminator
  Wind-axes Velocities : Subsystem
  body_rates_adim : Product  Inputs=/*
  AeroCoeff_b : Outport
  qbar (pdyn) : Outport  Port=2
  VBetaAlpha : Outport  Port=3
  wires:
  Vb_dot/1 -> Wind-axes Velocities/5(Vb_dot)
  V_Wind_b/1 -> Wind-axes Velocities/2(V_wind_b)
  Mux/1 -> AeroCoeff_b/1
  rho/1 -> Wind-axes Velocities/4(rho)
  Vb/1 -> Wind-axes Velocities/1(Vb)
  "a "/1 -> Wind-axes Velocities/3(a)  "speed of sound"
  omega_b/1 -> Sum/1
  Wind_omega_b/1 -> Sum/2
  Sum/1 -> Gain/1  "pqr"
  Sups_control_rad/1 -> Deflex mixer/1(Sups_control)
  Gain/1 -> body_rates_adim/2
  Wind-axes Velocities/5(TAS) -> Gain1/1, Mux2/1
  Gain1/1 -> body_rates_adim/1
  Deflex mixer/1(delta_ail_Asim) -> Mux1/1
  Deflex mixer/2(delta_rv_sim) -> Mux1/2
  Deflex mixer/3(delta_rv_Asim) -> Mux1/3
  Wind-axes Velocities/3(alpha) -> Mux2/3, Force Coefficients/1(alpha), Moment Coefficients/1(alpha)
  body_rates_adim/1 -> Force Coefficients/3(body_rates_adim), Moment Coefficients/3(body_rates_adim)
  Mux1/1 -> Force Coefficients/4(defl_control), Moment Coefficients/4(defl_control)
  Wind-axes Velocities/4(beta) -> Mux2/2, Force Coefficients/2(beta), Moment Coefficients/2(beta)
  Force Coefficients/1("[C_X_T, C_Y_T, C_Z_T]") -> Mux/1
  Moment Coefficients/1("[C_l_T, C_m_T, C_n_T]") -> Mux/2
  Wind-axes Velocities/1(qbar (pdyn)) -> qbar (pdyn)/1
  Wind-axes Velocities/2(alphadot) -> Terminator/1
  Mux2/1 -> VBetaAlpha/1

== system DBX_model_all/aeromodel/Aero model/Wind Model ==
  note: Wind Models
  Alt (m) : Inport
  DCM : Inport  Port=2
  V_e (m/s) : Inport  Port=3
  Dot Product : DotProduct  SaturateOnIntegerOverflow=on  OutDataTypeStr=Inherit: Inherit via internal rule
  Dryden Wind Turbulence Model (Continuous (+q +r)) : aerolibwind2/Dryden Wind Turbulence Model  (Continuous (+q -r))  units=Metric (MKS)  spec=MIL-F-8785C  model=Continuous Von Karman (+q -r)  W20=0  Wdeg=90  TurbProb=2x10^-1  L_high=533.4  Wingspan=B_span  ts=0.02  Seed=[23341 23342 23343 23344]  T_on=on
  Horizontal Wind Model : aerolibwind2/Horizontal Wind Model  units=Metric (MKS)  Vw_source=Internal  Vwind=0  W_source=Internal  Wdeg=-60
  Sum : Sum  Inputs=+++  SaturateOnIntegerOverflow=on  InputSameDT=on  OutDataTypeStr=Inherit: Same as first input
  V : Math  Operator=sqrt  SaturateOnIntegerOverflow=on
  Wind Shear Model : aerolibwind2/Wind Shear Model  units=Metric (MKS)  phase=Category C - Terminal Flight Phase  W_20=0  Wdeg=0
  V_wind : Outport
  omega_wind : Outport  Port=2
  wires:
  V/1 -> Dryden Wind Turbulence Model (Continuous (+q +r))/2
  Dryden Wind Turbulence Model (Continuous (+q +r))/1 -> Sum/3
  V_e (m/s)/1 -> Dot Product/2, Dot Product/1
  Dot Product/1 -> V/1
  Dryden Wind Turbulence Model (Continuous (+q +r))/2 -> omega_wind/1
  Sum/1 -> V_wind/1
  DCM/1 -> Horizontal Wind Model/1, Dryden Wind Turbulence Model (Continuous (+q +r))/3, Wind Shear Model/2
  Alt (m)/1 -> Dryden Wind Turbulence Model (Continuous (+q +r))/1, Wind Shear Model/1
  Horizontal Wind Model/1 -> Sum/2
  Wind Shear Model/1 -> Sum/1

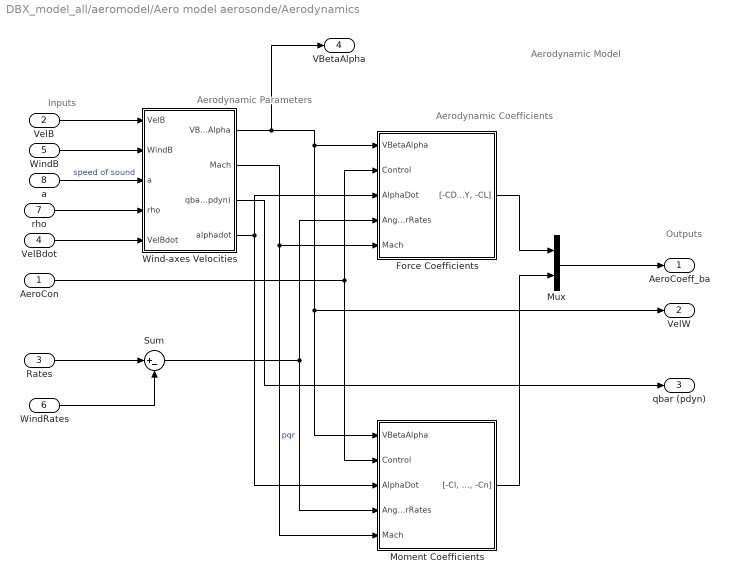
== system DBX_model_all/aeromodel/Aero model aerosonde/Aerodynamics ==
  note: Aerodynamic Model
  note: Aerodynamic Coefficients
  note: Aerodynamic Parameters
  note: Outputs
  note: Inputs
  AeroCon : Inport  PortDimensions=[4 1]
  VelB : Inport  Port=2  PortDimensions=[3 1]
  Rates : Inport  Port=3  PortDimensions=[3 1]
  VelBdot : Inport  Port=4
  WindB : Inport  Port=5  PortDimensions=[3 1]
  WindRates : Inport  Port=6  PortDimensions=[3 1]
  rho : Inport  Port=7  PortDimensions=1
  "a " : Inport  Port=8  PortDimensions=1
  Force Coefficients : Subsystem
  Moment Coefficients : Subsystem
  Mux : Mux  Inputs=2
  Sum : Sum  Inputs=|+-  SaturateOnIntegerOverflow=on  InputSameDT=on  OutDataTypeStr=Inherit: Same as first input
  Wind-axes Velocities : Subsystem
  AeroCoeff_ba : Outport
  VelW : Outport  Port=2
  qbar (pdyn) : Outport  Port=3
  VBetaAlpha : Outport  Port=4
  wires:
  VelBdot/1 -> Wind-axes Velocities/5(VelBdot)
  Wind-axes Velocities/4(alphadot) -> Force Coefficients/3(AlphaDot), Moment Coefficients/3(AlphaDot)
  WindB/1 -> Wind-axes Velocities/2(WindB)
  Mux/1 -> AeroCoeff_ba/1
  Moment Coefficients/1("[-Cl, Cm, -Cn]") -> Mux/2
  Force Coefficients/1("[-CD, CY, -CL]") -> Mux/1
  rho/1 -> Wind-axes Velocities/4(rho)
  VelB/1 -> Wind-axes Velocities/1(VelB)
  "a "/1 -> Wind-axes Velocities/3(a)  "speed of sound"
  AeroCon/1 -> Moment Coefficients/2(Control), Force Coefficients/2(Control)
  Wind-axes Velocities/2(Mach) -> Moment Coefficients/5(Mach), Force Coefficients/5(Mach)
  Wind-axes Velocities/3(qbar (pdyn)) -> qbar (pdyn)/1
  Rates/1 -> Sum/1
  WindRates/1 -> Sum/2
  Sum/1 -> Moment Coefficients/4(AngularRates), Force Coefficients/4(AngularRates)  "pqr"
  Wind-axes Velocities/1(VBetaAlpha) -> VBetaAlpha/1, Moment Coefficients/1(VBetaAlpha), VelW/1, Force Coefficients/1(VBetaAlpha)

== system DBX_model_all/aeromodel/Aero model aerosonde/Deflex mixer ==
  note: Control inputs:
      |
      |
      | 7. Rudervator Left (rad)
      | 8. Rudervator Right (rad)
      | 9. Aileron Left (rad)
      | 10. Aielron Right (rad)
  Sups_control : Inport
  Add : Sum  Inputs=|+-
  Add1 : Sum  Inputs=|++
  Add2 : Sum  Inputs=|+-
  Demux : Demux
  Gain : Gain  Gain=1/2
  Gain1 : Gain  Gain=1/2
  Gain2 : Gain  Gain=1/2
  delta_ail_Asim : Outport
  delta_rv_sim : Outport  Port=2
  delta_rv_Asim : Outport  Port=3
  wires:
  Sups_control/1 -> Demux/1
  Demux/3 -> Add/1
  Demux/4 -> Add/2
  Add/1 -> Gain/1
  Gain/1 -> delta_ail_Asim/1
  Demux/1 -> Add2/1, Add1/1
  Demux/2 -> Add2/2, Add1/2
  Add2/1 -> Gain1/1
  Add1/1 -> Gain2/1
  Gain2/1 -> delta_rv_sim/1
  Gain1/1 -> delta_rv_Asim/1

== system DBX_model_all/aeromodel/Aero model aerosonde/Wind Model ==
  note: Wind Models
  Alt (m) : Inport
  DCM : Inport  Port=2
  V_e (m/s) : Inport  Port=3
  Dot Product : DotProduct  SaturateOnIntegerOverflow=on  OutDataTypeStr=Inherit: Inherit via internal rule
  Dryden Wind Turbulence Model (Continuous (+q +r)) : aerolibwind2/Dryden Wind Turbulence Model  (Continuous (+q -r))  units=Metric (MKS)  spec=MIL-F-8785C  model=Continuous Von Karman (+q -r)  W20=0  Wdeg=90  TurbProb=2x10^-1  L_high=533.4  Wingspan=B_span  ts=0.02  Seed=[23341 23342 23343 23344]  T_on=on
  Horizontal Wind Model : aerolibwind2/Horizontal Wind Model  units=Metric (MKS)  Vw_source=Internal  Vwind=0  W_source=Internal  Wdeg=-60
  Sum : Sum  Inputs=+++  SaturateOnIntegerOverflow=on  InputSameDT=on  OutDataTypeStr=Inherit: Same as first input
  V : Math  Operator=sqrt  SaturateOnIntegerOverflow=on
  Wind Shear Model : aerolibwind2/Wind Shear Model  units=Metric (MKS)  phase=Category C - Terminal Flight Phase  W_20=0  Wdeg=0
  V_wind : Outport
  omega_wind : Outport  Port=2
  wires:
  V/1 -> Dryden Wind Turbulence Model (Continuous (+q +r))/2
  Dryden Wind Turbulence Model (Continuous (+q +r))/1 -> Sum/3
  V_e (m/s)/1 -> Dot Product/2, Dot Product/1
  Dot Product/1 -> V/1
  Dryden Wind Turbulence Model (Continuous (+q +r))/2 -> omega_wind/1
  Sum/1 -> V_wind/1
  DCM/1 -> Horizontal Wind Model/1, Dryden Wind Turbulence Model (Continuous (+q +r))/3, Wind Shear Model/2
  Alt (m)/1 -> Dryden Wind Turbulence Model (Continuous (+q +r))/1, Wind Shear Model/1
  Horizontal Wind Model/1 -> Sum/2
  Wind Shear Model/1 -> Sum/1

== system DBX_model_all/aeromodel/Aero model/Aerodynamics/Deflex mixer ==
  note: Control inputs:
      |
      |
      | 7. Rudervator Left (rad)
      | 8. Rudervator Right (rad)
      | 9. Aileron Left (rad)
      | 10. Aielron Right (rad)
  Sups_control : Inport
  Add : Sum  Inputs=|+-
  Add1 : Sum  Inputs=|++
  Add2 : Sum  Inputs=|+-
  Demux : Demux
  Gain : Gain  Gain=1/2
  Gain1 : Gain  Gain=1/2
  Gain2 : Gain  Gain=1/2
  delta_ail_Asim : Outport
  delta_rv_sim : Outport  Port=2
  delta_rv_Asim : Outport  Port=3
  wires:
  Sups_control/1 -> Demux/1
  Demux/3 -> Add/1
  Demux/4 -> Add/2
  Add/1 -> Gain/1
  Gain/1 -> delta_ail_Asim/1
  Demux/1 -> Add2/1, Add1/1
  Demux/2 -> Add2/2, Add1/2
  Add2/1 -> Gain1/1
  Add1/1 -> Gain2/1
  Gain2/1 -> delta_rv_sim/1
  Gain1/1 -> delta_rv_Asim/1

== system DBX_model_all/aeromodel/Aero model/Aerodynamics/Force Coefficients ==
  note: Con Cariño para Luis :P
  note: Deflexiones efectivas:
      |
      | delta_ail_Asim
      | delta_rv_sim
      | delta_rv_Asim
  alpha : Inport
  beta : Inport  Port=2
  body_rates_adim : Inport  Port=3
  defl_control : Inport  Port=4
  C_X_T : Subsystem
  C_Y_T : Subsystem
  C_Z_T : Subsystem
  Mux : Mux  Inputs=3
  "[C_X_T, C_Y_T, C_Z_T]" : Outport
  wires:
  alpha/1 -> C_Z_T/1(alpha), C_Y_T/1(alpha), C_X_T/1(alpha)
  beta/1 -> C_Z_T/2(beta), C_Y_T/2(beta), C_X_T/2(beta)
  body_rates_adim/1 -> C_Z_T/3(body_rates_adim), C_Y_T/3(body_rates_adim), C_X_T/3(body_rates_adim)
  defl_control/1 -> C_Z_T/4(defl_control), C_Y_T/4(defl_control), C_X_T/4(defl_control)
  C_Y_T/1(C_Y_T) -> Mux/2
  Mux/1 -> "[C_X_T, C_Y_T, C_Z_T]"/1
  C_X_T/1(C_X_T) -> Mux/1
  C_Z_T/1(C_Z_T) -> Mux/3

== system DBX_model_all/aeromodel/Aero model/Aerodynamics/Moment Coefficients ==
  note: Con Cariño para Luis :P
  note: Deflexiones efectivas:
      |
      | delta_ail_Asim
      | delta_rv_sim
      | delta_rv_Asim
  alpha : Inport
  beta : Inport  Port=2
  body_rates_adim : Inport  Port=3  PortDimensions=[3 1]
  defl_control : Inport  Port=4
  C_l_T : Subsystem
  C_m_T : Subsystem
  C_n_T : Subsystem
  Mux : Mux  Inputs=3
  "[C_l_T, C_m_T, C_n_T]" : Outport
  wires:
  alpha/1 -> C_n_T/1(alpha), C_m_T/1(alpha), C_l_T/1(alpha)
  beta/1 -> C_n_T/2(beta), C_m_T/2(beta), C_l_T/2(beta)
  body_rates_adim/1 -> C_n_T/3(body_rates_adim), C_m_T/3(body_rates_adim), C_l_T/3(body_rates_adim)
  defl_control/1 -> C_n_T/4(defl_control), C_m_T/4(defl_control), C_l_T/4(defl_control)
  Mux/1 -> "[C_l_T, C_m_T, C_n_T]"/1
  C_l_T/1(C_l_T) -> Mux/1
  C_m_T/1(C_m_T) -> Mux/2
  C_n_T/1(C_n_T) -> Mux/3

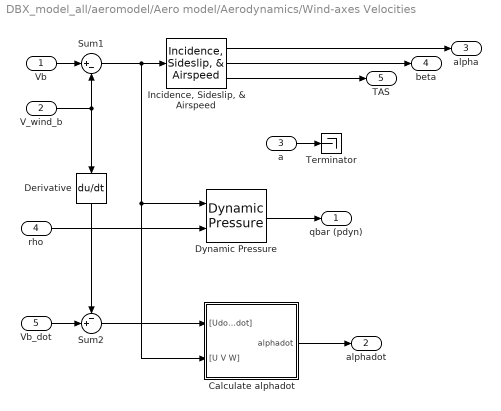
== system DBX_model_all/aeromodel/Aero model/Aerodynamics/Wind-axes Velocities ==
  Vb : Inport
  V_wind_b : Inport  Port=2
  a : Inport  Port=3
  rho : Inport  Port=4
  Vb_dot : Inport  Port=5
  Calculate alphadot : Subsystem
  Derivative : Derivative  CoefficientInTFapproximation=500
  Dynamic Pressure : aerolibasang/Dynamic Pressure
  "Incidence, Sideslip, & Airspeed" : aerolibasang/Incidence, Sideslip, & Airspeed
  Sum1 : Sum  Inputs=|+-  SaturateOnIntegerOverflow=on  InputSameDT=on  OutDataTypeStr=Inherit: Same as first input
  Sum2 : Sum  Inputs=-+|  SaturateOnIntegerOverflow=on  InputSameDT=on  OutDataTypeStr=Inherit: Same as first input
  Terminator : Terminator
  qbar (pdyn) : Outport
  alphadot : Outport  Port=2
  alpha : Outport  Port=3
  beta : Outport  Port=4
  TAS : Outport  Port=5
  wires:
  Derivative/1 -> Sum2/1
  Sum2/1 -> Calculate alphadot/1("[Udot Vdot Wdot]")
  Vb_dot/1 -> Sum2/2
  Calculate alphadot/1(alphadot) -> alphadot/1
  Dynamic Pressure/1 -> qbar (pdyn)/1
  rho/1 -> Dynamic Pressure/2
  V_wind_b/1 -> Derivative/1, Sum1/2
  Vb/1 -> Sum1/1
  Sum1/1 -> Calculate alphadot/2("[U V W]"), Dynamic Pressure/1, "Incidence, Sideslip, & Airspeed"/1
  "Incidence, Sideslip, & Airspeed"/3 -> TAS/1
  "Incidence, Sideslip, & Airspeed"/2 -> beta/1
  "Incidence, Sideslip, & Airspeed"/1 -> alpha/1
  a/1 -> Terminator/1

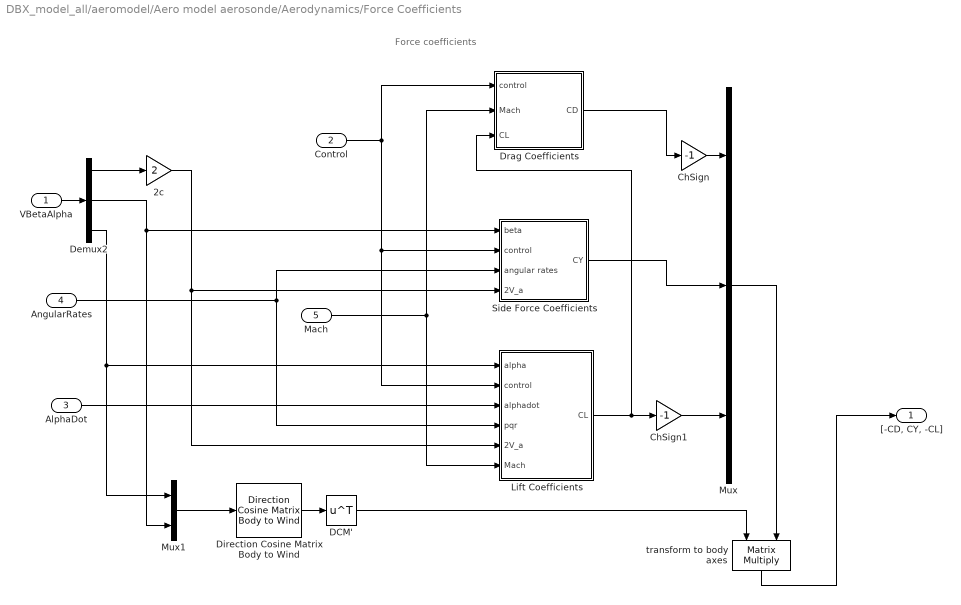
== system DBX_model_all/aeromodel/Aero model aerosonde/Aerodynamics/Force Coefficients ==
  note: Force coefficients
  VBetaAlpha : Inport  PortDimensions=[3 1]
  Control : Inport  Port=2  PortDimensions=[4 1]
  AlphaDot : Inport  Port=3
  AngularRates : Inport  Port=4  PortDimensions=[3 1]
  Mach : Inport  Port=5  PortDimensions=1
  2c : Gain  Gain=2  SaturateOnIntegerOverflow=on  OutDataTypeStr=Inherit: Same as input  ParamDataTypeStr=Inherit: Same as input
  ChSign : Gain  Gain=-1  SaturateOnIntegerOverflow=on  OutDataTypeStr=Inherit: Same as input  ParamDataTypeStr=Inherit: Same as input
  ChSign1 : Gain  Gain=-1  SaturateOnIntegerOverflow=on  OutDataTypeStr=Inherit: Same as input  ParamDataTypeStr=Inherit: Same as input
  DCM' : Math  Operator=transpose  SaturateOnIntegerOverflow=on
  Demux2 : Demux  Outputs=3
  Direction Cosine Matrix Body to Wind : aerolibtransform2/Direction Cosine Matrix Body to Wind
  Drag Coefficients : Subsystem
  Lift Coefficients : Subsystem
  Mux : Mux  Inputs=3
  Mux1 : Mux  Inputs=2
  Side Force Coefficients : Subsystem
  transform to body axes : Product  Inputs=**  Multiplication=Matrix(*)  SaturateOnIntegerOverflow=on  InputSameDT=on  OutDataTypeStr=Inherit: Same as first input
  "[-CD, CY, -CL]" : Outport
  wires:
  Mux1/1 -> Direction Cosine Matrix Body to Wind/1
  DCM'/1 -> transform to body axes/1
  Mux/1 -> transform to body axes/2
  Direction Cosine Matrix Body to Wind/1 -> DCM'/1
  transform to body axes/1 -> "[-CD, CY, -CL]"/1
  Demux2/2 -> Mux1/2, Side Force Coefficients/1(beta)
  Demux2/1 -> 2c/1
  VBetaAlpha/1 -> Demux2/1
  ChSign1/1 -> Mux/3
  ChSign/1 -> Mux/1
  Side Force Coefficients/1(CY) -> Mux/2
  Drag Coefficients/1(CD) -> ChSign/1
  Lift Coefficients/1(CL) -> Drag Coefficients/3(CL), ChSign1/1
  Mach/1 -> Drag Coefficients/2(Mach), Lift Coefficients/6(Mach)
  AngularRates/1 -> Side Force Coefficients/3(angular rates), Lift Coefficients/4(pqr)
  AlphaDot/1 -> Lift Coefficients/3(alphadot)
  Control/1 -> Side Force Coefficients/2(control), Lift Coefficients/2(control), Drag Coefficients/1(control)
  Demux2/3 -> Lift Coefficients/1(alpha), Mux1/1
  2c/1 -> Side Force Coefficients/4(2V_a), Lift Coefficients/5(2V_a)

== system DBX_model_all/aeromodel/Aero model aerosonde/Aerodynamics/Moment Coefficients ==
  note: Moment coefficients
  VBetaAlpha : Inport  PortDimensions=[3 1]
  Control : Inport  Port=2  PortDimensions=[4 1]
  AlphaDot : Inport  Port=3
  AngularRates : Inport  Port=4  PortDimensions=[3 1]
  Mach : Inport  Port=5  PortDimensions=1
  2c : Gain  Gain=2  SaturateOnIntegerOverflow=on  OutDataTypeStr=Inherit: Same as input  ParamDataTypeStr=Inherit: Same as input
  Demux1 : Demux  Outputs=3
  Mux : Mux  Inputs=3
  Pitch Moment Coefficients : Subsystem
  Roll Moment Coefficients : Subsystem
  Yaw Moment Coefficients : Subsystem
  "[-Cl, Cm, -Cn]" : Outport
  wires:
  Demux1/2 -> Yaw Moment Coefficients/1(beta), Roll Moment Coefficients/1(beta)
  Demux1/3 -> Pitch Moment Coefficients/1(alpha)
  Mach/1 -> Pitch Moment Coefficients/6(Mach)
  Yaw Moment Coefficients/1(Cn) -> Mux/3
  VBetaAlpha/1 -> Demux1/1
  2c/1 -> Pitch Moment Coefficients/5(2V_a), Yaw Moment Coefficients/4(2V_a), Roll Moment Coefficients/4(2V)
  Demux1/1 -> 2c/1
  Control/1 -> Yaw Moment Coefficients/2(control), Pitch Moment Coefficients/2(control), Roll Moment Coefficients/2(control)
  AlphaDot/1 -> Pitch Moment Coefficients/3(alphadot)
  AngularRates/1 -> Roll Moment Coefficients/3(angular rates), Yaw Moment Coefficients/3(angular rates), Pitch Moment Coefficients/4(pqr)
  Mux/1 -> "[-Cl, Cm, -Cn]"/1
  Pitch Moment Coefficients/1(Cm) -> Mux/2
  Roll Moment Coefficients/1(Cl) -> Mux/1

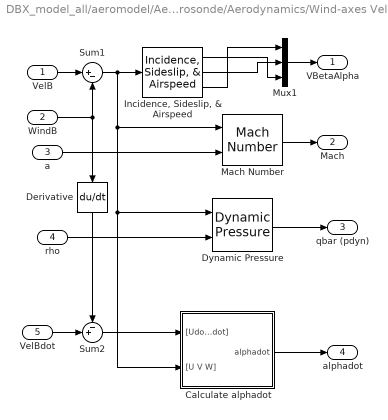
== system DBX_model_all/aeromodel/Aero model aerosonde/Aerodynamics/Wind-axes Velocities ==
  VelB : Inport
  WindB : Inport  Port=2
  a : Inport  Port=3
  rho : Inport  Port=4
  VelBdot : Inport  Port=5
  Calculate alphadot : Subsystem
  Derivative : Derivative
  Dynamic Pressure : aerolibasang/Dynamic Pressure
  "Incidence, Sideslip, & Airspeed" : aerolibasang/Incidence, Sideslip, & Airspeed
  Mach Number : aerolibasang/Mach Number
  Mux1 : Mux  Inputs=3
  Sum1 : Sum  Inputs=|+-  SaturateOnIntegerOverflow=on  InputSameDT=on  OutDataTypeStr=Inherit: Same as first input
  Sum2 : Sum  Inputs=-+|  SaturateOnIntegerOverflow=on  InputSameDT=on  OutDataTypeStr=Inherit: Same as first input
  VBetaAlpha : Outport
  Mach : Outport  Port=2
  qbar (pdyn) : Outport  Port=3
  alphadot : Outport  Port=4
  wires:
  Derivative/1 -> Sum2/1
  Sum2/1 -> Calculate alphadot/1("[Udot Vdot Wdot]")
  VelBdot/1 -> Sum2/2
  Calculate alphadot/1(alphadot) -> alphadot/1
  "Incidence, Sideslip, & Airspeed"/2 -> Mux1/2
  "Incidence, Sideslip, & Airspeed"/1 -> Mux1/3
  Dynamic Pressure/1 -> qbar (pdyn)/1
  rho/1 -> Dynamic Pressure/2
  a/1 -> Mach Number/2
  Mach Number/1 -> Mach/1
  WindB/1 -> Derivative/1, Sum1/2
  VelB/1 -> Sum1/1
  Mux1/1 -> VBetaAlpha/1
  "Incidence, Sideslip, & Airspeed"/3 -> Mux1/1
  Sum1/1 -> Calculate alphadot/2("[U V W]"), Dynamic Pressure/1, Mach Number/1, "Incidence, Sideslip, & Airspeed"/1

== system DBX_model_all/aeromodel/Aero model/Aerodynamics/Force Coefficients/C_X_T ==
  note: Deflexiones efectivas:
      |
      | delta_ail_Asim
      | delta_rv_sim
      | delta_rv_Asim
  alpha : Inport
  beta : Inport  Port=2
  body_rates_adim : Inport  Port=3  PortDimensions=[3 1]
  defl_control : Inport  Port=4
  Add : Sum  Inputs=++|
  Add1 : Sum  Inputs=-+|
  C_D_q : Constant  Value=C_D_q
  C_Lift_q : Constant  Value=C_Lift_q
  C_X : Lookup_n-D  NumberOfTableDimensions=3  BreakpointsForDimension1=Alpha_unique_rad  BreakpointsForDimension2=Beta_unique_rad  BreakpointsForDimension3=delta_elev_unique_rad  Table=C_X  DiagnosticForOutOfRangeInput=Warning  RemoveProtectionInput=on  InternalRulePriority=Speed  RndMeth=Simplest  InputSameDT=on
  Divide : Product  Inputs=**
  Divide1 : Product  Inputs=**
  Divide2 : Product  Inputs=**
  Selector : Selector  InputPortWidth=3  Indices=2
  Selector1 : Selector  InputPortWidth=3  Indices=2
  cos : Trigonometry  Operator=cos
  sin : Trigonometry
  C_X_T : Outport
  wires:
  alpha/1 -> cos/1, sin/1, C_X/1
  beta/1 -> C_X/2
  body_rates_adim/1 -> Selector/1
  Selector/1 -> Divide/1
  C_X/1 -> Add/1
  Divide/1 -> Add/2
  Add/1 -> C_X_T/1
  defl_control/1 -> Selector1/1
  Selector1/1 -> C_X/3
  sin/1 -> Divide1/1
  C_Lift_q/1 -> Divide1/2
  cos/1 -> Divide2/1
  C_D_q/1 -> Divide2/2
  Divide1/1 -> Add1/2
  Divide2/1 -> Add1/1
  Add1/1 -> Divide/2

== system DBX_model_all/aeromodel/Aero model/Aerodynamics/Force Coefficients/C_Y_T ==
  note: Deflexiones efectivas:
      |
      | delta_ail_Asim
      | delta_rv_sim
      | delta_rv_Asim
  alpha : Inport
  beta : Inport  Port=2
  body_rates_adim : Inport  Port=3  PortDimensions=[3 1]
  defl_control : Inport  Port=4
  Add : Sum  Inputs=++++
  C_Y : Lookup_n-D  BreakpointsForDimension1=Alpha_unique_rad  BreakpointsForDimension2=Beta_unique_rad  Table=C_Y  DiagnosticForOutOfRangeInput=Warning  RemoveProtectionInput=on  InternalRulePriority=Speed  RndMeth=Simplest  InputSameDT=on
  C_Y_delta_rv : Constant  Value=C_Y_delta_rv_Asim
  C_Y_p : Constant  Value=C_Y_p
  C_Y_r : Constant  Value=C_Y_r
  Divide : Product  Inputs=**
  Divide1 : Product  Inputs=**
  Divide2 : Product  Inputs=**
  Selector : Selector  InputPortWidth=3  Indices=3
  Selector1 : Selector  InputPortWidth=3
  Selector2 : Selector  InputPortWidth=3  Indices=3
  C_Y_T : Outport
  wires:
  alpha/1 -> C_Y/1
  beta/1 -> C_Y/2
  Selector/1 -> Divide/1
  C_Y_r/1 -> Divide/2
  body_rates_adim/1 -> Selector1/1, Selector/1
  Selector1/1 -> Divide1/1
  C_Y_p/1 -> Divide1/2
  defl_control/1 -> Selector2/1
  C_Y_delta_rv/1 -> Divide2/2
  Selector2/1 -> Divide2/1
  Divide2/1 -> Add/4
  Divide1/1 -> Add/3
  Divide/1 -> Add/2
  C_Y/1 -> Add/1
  Add/1 -> C_Y_T/1
